simulink model "gm_interleaver_model"  (R2020b)
settings: Solver=FixedStepDiscrete  StartTime=0.0  StopTime=30  RelTol=1e-3
libraries: commdigbbndpm3 x1, commrandsrc3 x1
settings Model: Creator=wardo  LastModifiedBy=wardo
settings DataIOCC: LimitDataPoints=on  SaveOutput=off  SaveTime=off
settings OptimizationCC: BlockReduction=off  ConditionallyExecuteInputs=off  DefaultParameterBehavior=Inlined  LifeSpan=inf
settings DebuggingCC: AlgebraicLoopMsg=error  InheritedTsInSrcMsg=none  SingleTaskRateTransMsg=error  AllowSymbolicDim=off  StrictBusMsg=ErrorOnBusTreatedAsVector  SFUnexpectedBacktrackingDiag=warning  SFNoUnconditionalDefaultTransitionDiag=warning  SFExecutionAtInitializationDiag=none  ArithmeticOperatorsInVariantConditions=warning
settings HardwareCC: ProdBitPerPointer=32  ProdBitPerSizeT=32  ProdBitPerPtrDiffT=32  ProdLargestAtomicFloat=None  ProdIntDivRoundTo=Undefined  ProdEndianess=Unspecified  ProdWordSize=32  ProdHWDeviceType=ASIC/FPGA->ASIC/FPGA  ProdEqTarget=off
settings SFSimCC: SimUseLocalCustomCode=off  CustomCodeUndefinedFunction=UseInterfaceOnly
settings RTWCC: RTWUseLocalCustomCode=off
settings CodeAppCC: StateflowObjectComments=on
settings GRTTargetCC: TargetLangStandard=C89/C90 (ANSI)
settings ConfigComp: CovScope=ReferencedModels  CovMetricSettings=dw  CovSaveCumulativeToWorkspaceVar=on  CovSaveSingleToWorkspaceVar=on  CovExternalEMLEnable=off  CovSFcnEnable=off

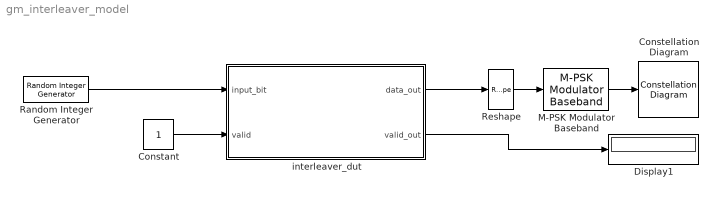
== system gm_interleaver_model ==
  Constant : Constant  OutDataTypeStr=boolean  SampleTime=-1
  Constellation Diagram : ConstellationDiagram
  Display1 : Display
  M-PSK Modulator Baseband : commdigbbndpm3/M-PSK Modulator Baseband  M=8  InType=Bit  Enc=Gray  Mapping=[0:7]  Ph=0  outDtype=double  outWordLen=16  outUDDataType=sfix(16)  outFracLenMode=Best precision  outFracLen=15  outDataTypeStr=double  outLastDataTypeStr=double
      settings: SourceProductName=Communications Toolbox
  Random Integer Generator : commrandsrc3/Random Integer Generator  SetSize=2  SeedSource=Auto  Seed=0  SampleTime=1  SamplesPerFrame=1  OutputDataType=boolean  SimulateUsing=Interpreted execution
  Reshape : Reshape
  interleaver_dut : Subsystem
  wires:
  Reshape/1 -> M-PSK Modulator Baseband/1
  M-PSK Modulator Baseband/1 -> Constellation Diagram/1
  interleaver_dut/1(data_out) -> Reshape/1
  interleaver_dut/2(valid_out) -> Display1/1
  Constant/1 -> interleaver_dut/2(valid)
  Random Integer Generator/1 -> interleaver_dut/1(input_bit)

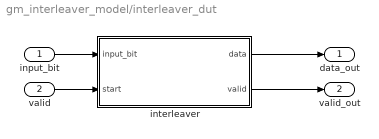
== system gm_interleaver_model/interleaver_dut ==
  input_bit : Inport
  valid : Inport  Port=2
  interleaver : MATLAB Function  TreatAsAtomicUnit=on
  data_out : Outport  VectorParamsAs1DForOutWhenUnconnected=off
  valid_out : Outport  Port=2  VectorParamsAs1DForOutWhenUnconnected=off
  wires:
  interleaver/2(valid) -> valid_out/1
  interleaver/1(data) -> data_out/1
  valid/1 -> interleaver/2(start)
  input_bit/1 -> interleaver/1(input_bit)

== matlab function gm_interleaver_model/interleaver_dut/interleaver ==
  settings: fimath=fimath('RoundingMethod', 'Floor','OverflowAction', 'Wrap','ProductMode', 'FullPrecision', 'SumMode', 'FullPrecision')
  data: input_bit input; data output; start input; valid output
function [data, valid] = fsm_interleaver(input_bit, start)
%#codegen

rows           = 4;
columns        = 3;
state_iddle    = 0;
state_writting = 1;
state_reading  = 2;

persistent moore_state_reg;
if isempty(moore_state_reg)
    moore_state_reg = fi(0, 0, 2, 0);   
end

persistent counter;
if isempty(counter)
    counter = fi(1, 0, 16, 0);
end

persistent column;
if isempty(column)
    column = fi(1, 0, 8, 0);   
end

persistent buffer;
if isempty(buffer)
    buffer = fi(zeros(rows, columns), 0, 1, 0);
end

switch (moore_state_reg)
    
    case state_iddle
        counter = fi(1, 0, 16, 0);   
        column  = fi(1, 0, 8, 0);   
        buffer  = fi(zeros(rows, columns), 0, 1, 0);
        valid   = false;
        data    = fi([0 0 0], 0, 1, 0);
        if (~start)
            moore_state_reg(1) = state_iddle;
        else
            moore_state_reg(1) = state_writting;
            % Write first bit at the bottom-rightest bit of the buffer
            buffer(rows - counter + 1, columns - column + 1) = input_bit;
            counter = fi(counter + 1, 0, 16, 0);
        end
        
    case state_writting
        buffer(rows - counter + 1, columns - column + 1) = input_bit;
        counter = fi(counter + 1, 0, 16, 0);
        if counter > rows
            counter = fi(1, 0, 16, 0);
            column  = fi(column + 1, 0, 8, 0);
            if (column > columns)
                moore_state_reg(1) = state_reading;
                counter = fi(1, 0, 16, 0);   
                column  = fi(1, 0, 8, 0);   
                valid   = true;
                data    = buffer(counter, :);
                counter = fi(counter + 1, 0, 16, 0);
            else
                data    = fi([0 0 0], 0, 1, 0);
                valid   = false;
            end
        else
            valid   = false;
            data    = fi([0 0 0], 0, 1, 0);
        end
    case state_reading
        data = buffer(counter, :);
        counter = fi(counter + 1, 0, 16, 0);
        if counter > rows
            moore_state_reg(1) = state_iddle;
        end
        valid = true;
    otherwise
        valid = false;
        data  = fi([0 0 0], 0, 1, 0);
        
end
